simulink model "PID_PalmSat_mono"  (R2017b)
settings: Solver=VariableStepAuto  StartTime=0.0  StopTime=400  RelTol=1e-3
values from neighbouring files (symbols this model uses):
  B = ModeloSatelite.B    [PalmSatModelScript.m]
  IA = 6645861.83/10^9    (= 0.00664586183)    [PalmSatModelScript.m]
  IB = 12785011.68/(10^9)    (= 0.01278501168)    [PalmSatModelScript.m]
  IC = 6645861.83/10^9    (= 0.00664586183)    [PalmSatModelScript.m]
  J = Jm + Jr    (= 0.000179383)    [PalmSatModelScript.m]
  Kpx = 10    [PalmSatModelScript.m]
  Kpy = 10    [PalmSatModelScript.m]
  Kpz = Kc    [PalmSatModelScript.m]
  Kt = Kw/0.00684    (= 25.0525729951)    [PalmSatModelScript.m]
  Kw = 60*2*pi/2200    (= 0.171359599287)    [PalmSatModelScript.m]
  La = 74.4*10^-6    (= 7.44e-05)    [PalmSatModelScript.m]
  Ra = 0.225    [PalmSatModelScript.m]
  Tdx = 0    [PalmSatModelScript.m]
  Tdy = 0    [PalmSatModelScript.m]
  Tdz = Pu*0.125    (= 1.85)    [PalmSatModelScript.m]
  Tix = 10^10    (= 10000000000)    [PalmSatModelScript.m]
  Tiy = 10^10    (= 10000000000)    [PalmSatModelScript.m]
  Tiz = Pu*0.5    (= 7.4)    [PalmSatModelScript.m]
settings Model: Creator=Gpiaia  LastModifiedBy=Gpiaia
settings OptimizationCC: EfficientMapNaN2IntZero=off
settings HardwareCC: TargetBitPerPointer=64  TargetBitPerSizeT=64  TargetBitPerPtrDiffT=64  TargetLongLongMode=on  TargetIntDivRoundTo=Zero  TargetEndianess=LittleEndian  TargetWordSize=64  TargetHWDeviceType=MATLAB Host  ProdEqTarget=off
settings CodeAppCC: MaxIdLength=128
settings GRTTargetCC: TargetLangStandard=C89/C90 (ANSI)  CombineOutputUpdateFcns=off  GRTInterface=on

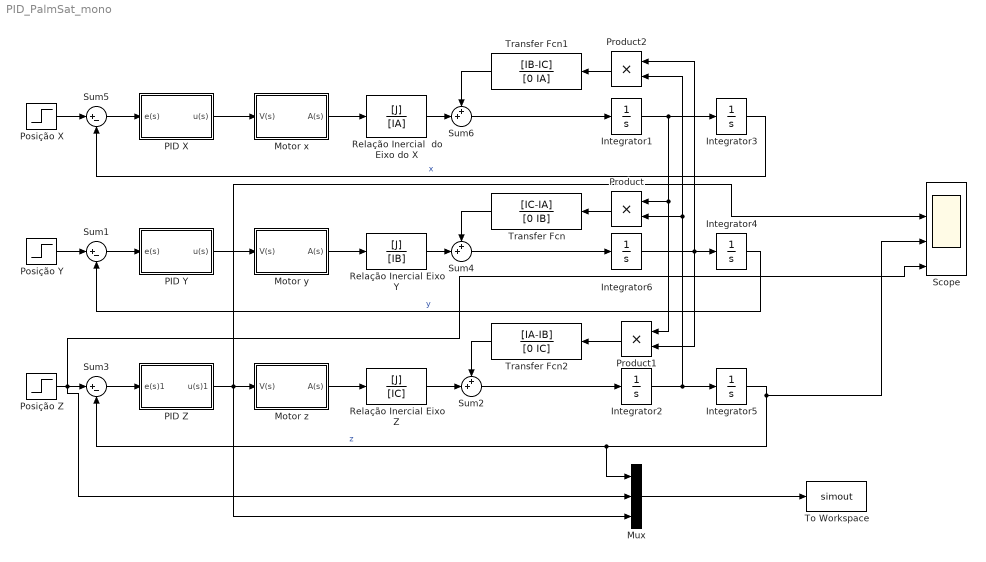
== system PID_PalmSat_mono ==
  Integrator{1..6} (6 alike) : Integrator
  Motor x : Subsystem
  Motor y : Subsystem
  Motor z : Subsystem
  Mux : Mux  Inputs=3
  PID X : Subsystem
  PID Y : Subsystem
  PID Z : Subsystem
  Posição X : Step  Time=5  After=0  SampleTime=0
  Posição Y : Step  Time=4  After=0  SampleTime=0
  Posição Z : Step  After=45  SampleTime=0
  Product : Product
  Product1 : Product
  Product2 : Product
  Relação Inercial Eixo Y : TransferFcn  Numerator=[J]  Denominator=[IB]
  Relação Inercial Eixo Z : TransferFcn  Numerator=[J]  Denominator=[IC]
  Relação Inercial  do Eixo do X : TransferFcn  Numerator=[J]  Denominator=[IA]
  Scope : Scope  NumInputPorts=4
  Sum1 : Sum  Inputs=|+-
  Sum2 : Sum  Inputs=++|
  Sum3 : Sum  Inputs=|+-
  Sum4 : Sum  Inputs=++|
  Sum5 : Sum  Inputs=|+-
  Sum6 : Sum  Inputs=++|
  To Workspace : ToWorkspace  VariableName=simout  SaveFormat=Timeseries  SampleTime=-1
  Transfer Fcn : TransferFcn  Numerator=[IC-IA]  Denominator=[0 IB]
  Transfer Fcn1 : TransferFcn  Numerator=[IB-IC]  Denominator=[0 IA]
  Transfer Fcn2 : TransferFcn  Numerator=[IA-IB]  Denominator=[0 IC]
  wires:
  Relação Inercial Eixo Y/1 -> Sum4/2
  Relação Inercial Eixo Z/1 -> Sum2/2
  Posição X/1 -> Sum5/1
  Transfer Fcn/1 -> Sum4/1
  Transfer Fcn2/1 -> Sum2/1
  Transfer Fcn1/1 -> Sum6/1
  Relação Inercial  do Eixo do X/1 -> Sum6/2
  Sum4/1 -> Integrator6/1
  Product1/1 -> Transfer Fcn2/1
  Integrator1/1 -> Integrator3/1, Product1/1, Product/1
  Integrator6/1 -> Integrator4/1, Product1/2, Product2/1
  Integrator5/1 -> Scope/3, Mux/1, Sum3/2  "z"
  Product2/1 -> Transfer Fcn1/1
  Posição Y/1 -> Sum1/1
  Integrator3/1 -> Sum5/2  "x"
  Integrator2/1 -> Integrator5/1, Product2/2, Product/2
  Product/1 -> Transfer Fcn/1
  Sum6/1 -> Integrator1/1
  Integrator4/1 -> Sum1/2  "y"
  Posição Z/1 -> Mux/2, Scope/4, Sum3/1
  Sum2/1 -> Integrator2/1
  Sum1/1 -> PID Y/1(e(s))
  Sum5/1 -> PID X/1(e(s))
  PID X/1(u(s)) -> Motor x/1(V(s))
  Motor x/1(A(s)) -> Relação Inercial  do Eixo do X/1
  Motor z/1(A(s)) -> Relação Inercial Eixo Z/1
  Motor y/1(A(s)) -> Relação Inercial Eixo Y/1
  PID Y/1(u(s)) -> Motor y/1(V(s))
  Mux/1 -> To Workspace/1
  PID Z/1(u(s)1) -> Scope/2, Mux/3, Motor z/1(V(s))
  Sum3/1 -> PID Z/1(e(s)1)

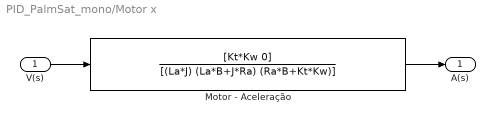
== system PID_PalmSat_mono/Motor x ==
  V(s) : Inport
  Motor - Aceleração : TransferFcn  Numerator=[Kt*Kw 0]  Denominator=[(La*J) (La*B+J*Ra) (Ra*B+Kt*Kw)]
  A(s) : Outport
  wires:
  V(s)/1 -> Motor - Aceleração/1
  Motor - Aceleração/1 -> A(s)/1

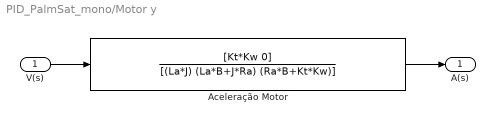
== system PID_PalmSat_mono/Motor y ==
  V(s) : Inport
  Aceleração Motor : TransferFcn  Numerator=[Kt*Kw 0]  Denominator=[(La*J) (La*B+J*Ra) (Ra*B+Kt*Kw)]
  A(s) : Outport
  wires:
  V(s)/1 -> Aceleração Motor/1
  Aceleração Motor/1 -> A(s)/1

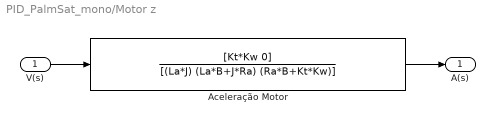
== system PID_PalmSat_mono/Motor z ==
  V(s) : Inport
  Aceleração Motor : TransferFcn  Numerator=[Kt*Kw 0]  Denominator=[(La*J) (La*B+J*Ra) (Ra*B+Kt*Kw)]  AbsoluteTolerance=1e-6
  A(s) : Outport
  wires:
  V(s)/1 -> Aceleração Motor/1
  Aceleração Motor/1 -> A(s)/1

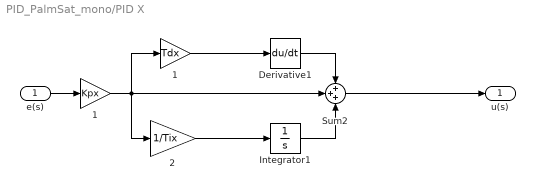
== system PID_PalmSat_mono/PID X ==
  e(s) : Inport
  " 1" : Gain  Gain=Tdx
  "  2" : Gain  Gain=1/Tix
  " 1" : Gain  Gain=Kpx
  Derivative1 : Derivative
  Integrator1 : Integrator
  Sum2 : Sum  Inputs=+++
  u(s) : Outport
  wires:
  " 1"/1 -> Derivative1/1
  " 1"/1 -> " 1"/1, Sum2/2, "  2"/1
  "  2"/1 -> Integrator1/1
  Sum2/1 -> u(s)/1
  Integrator1/1 -> Sum2/3
  Derivative1/1 -> Sum2/1
  e(s)/1 -> " 1"/1

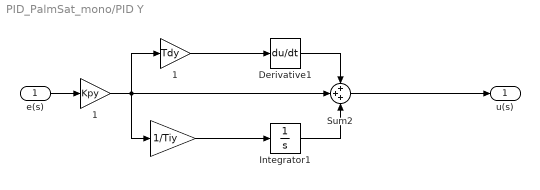
== system PID_PalmSat_mono/PID Y ==
  e(s) : Inport
  " 1" : Gain  Gain=Tdy
  "  " : Gain  Gain=1/Tiy
  " 1" : Gain  Gain=Kpy
  Derivative1 : Derivative
  Integrator1 : Integrator
  Sum2 : Sum  Inputs=+++
  u(s) : Outport
  wires:
  " 1"/1 -> Derivative1/1
  " 1"/1 -> " 1"/1, Sum2/2, "  "/1
  "  "/1 -> Integrator1/1
  Integrator1/1 -> Sum2/3
  Derivative1/1 -> Sum2/1
  e(s)/1 -> " 1"/1
  Sum2/1 -> u(s)/1

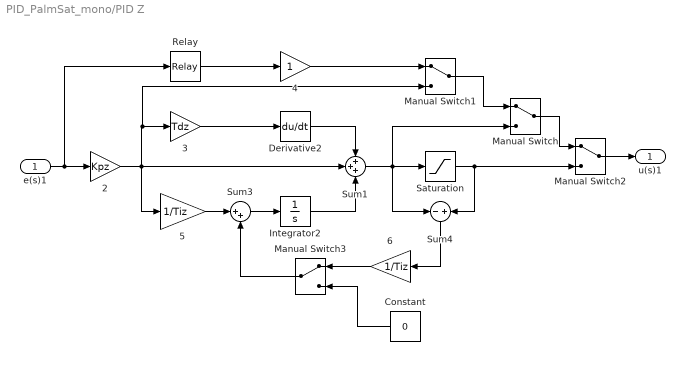
== system PID_PalmSat_mono/PID Z ==
  e(s)1 : Inport
  " 3" : Gain  Gain=Tdz
  " 4" : Gain
  "  5" : Gain  Gain=1/Tiz
  "  6" : Gain  Gain=1/Tiz
  " 2" : Gain  Gain=Kpz
  Constant : Constant  Value=0
  Derivative2 : Derivative
  Integrator2 : Integrator
  Manual Switch{,1..3} (4 alike) : ManualSwitch
  Relay : Relay  OnSwitchValue=+0.01  OffSwitchValue=-0.01  OnOutputValue=+1  OffOutputValue=-1
  Saturation : Saturate  UpperLimit=200  LowerLimit=-200
  Sum1 : Sum  Inputs=+++
  Sum3 : Sum  Inputs=|++
  Sum4 : Sum  Inputs=-+
  u(s)1 : Outport
  wires:
  " 2"/1 -> Manual Switch1/2, " 3"/1, Sum1/2, "  5"/1
  Manual Switch3/1 -> Sum3/2
  Manual Switch1/1 -> Manual Switch/1
  Sum4/1 -> "  6"/1
  Relay/1 -> " 4"/1
  Manual Switch2/1 -> u(s)1/1
  Sum1/1 -> Saturation/1, Manual Switch/2, Sum4/1
  " 4"/1 -> Manual Switch1/1
  Constant/1 -> Manual Switch3/2
  Manual Switch/1 -> Manual Switch2/1
  Derivative2/1 -> Sum1/1
  Integrator2/1 -> Sum1/3
  Saturation/1 -> Manual Switch2/2, Sum4/2
  e(s)1/1 -> Relay/1, " 2"/1
  Sum3/1 -> Integrator2/1
  "  5"/1 -> Sum3/1
  " 3"/1 -> Derivative2/1
  "  6"/1 -> Manual Switch3/1
